simulink model "SUPERCAPACITOR_closed_loop_boost"  (R2021a)
settings: Solver=VariableStepAuto  StartTime=0.0  StopTime=10.0  RelTol=1e-3
libraries: spsSeriesRLCBranchLib x7, spsMosfetLib x4, simulink x1, spsSupercapacitorLib x1, spsVoltageMeasurementLib x1, spspowerguiLib x1
settings Model: Creator=Bhargava  LastModifiedBy=Bhargava

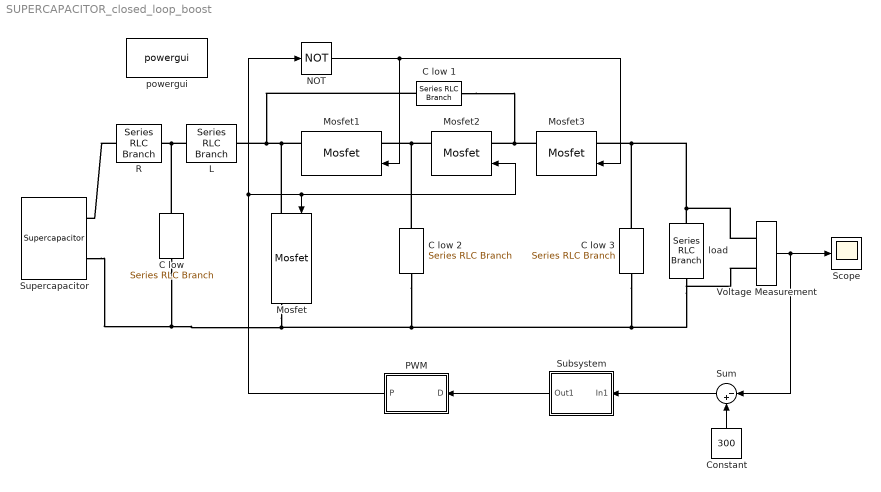
== system SUPERCAPACITOR_closed_loop_boost ==
  C low {,1..3} (4 alike) : spsSeriesRLCBranchLib/Series RLC Branch  LConnTagsString=__new0  RConnTagsString=__new0  BranchType=C  Resistance=1  Inductance=1e-3  SetiL0=off  InitialCurrent=0  Capacitance=520e-6  Setx0=off  InitialVoltage=0  Measurements=None
  Constant : Constant  Value=300
  L : spsSeriesRLCBranchLib/Series RLC Branch  LConnTagsString=__new0  RConnTagsString=__new0  BranchType=L  Resistance=1  Inductance=353e-3  SetiL0=off  InitialCurrent=0  Capacitance=1e-6  Setx0=off  InitialVoltage=0  Measurements=None
  Mosfet{,1..3} (4 alike) : spsMosfetLib/Mosfet  Ron=0.1  Lon=0  Rd=0.01  Vfd=0  IC=0  Rs=1e5  Cs=inf  Measurements=on
  NOT : Logic  Operator=NOT  IconShape=distinctive  AllPortsSameDT=off  OutDataTypeStr=boolean
  "PWM " : Subsystem
  R : spsSeriesRLCBranchLib/Series RLC Branch  LConnTagsString=__new0  RConnTagsString=__new0  BranchType=R  Resistance=0.0001  Inductance=1e-3  SetiL0=off  InitialCurrent=0  Capacitance=1e-6  Setx0=off  InitialVoltage=0  Measurements=None
  Scope : Scope
  Subsystem : Subsystem
  Sum : Sum  Inputs=|-+
  Supercapacitor : spsSupercapacitorLib/Supercapacitor  C=99.5  Rdc=8.9e-3  Voltage=200  Ns=18  Np=1  Vinit=45  Temp=25  PresetModel=off  EstParam=off  Nc=1  r=1e-9  epsilon=6.0208e-10  Ich=10  Vstern="[0.161  2.7  7.8]"  Self_dis=on  Ioc=10  Vself="[48  47.8  47.06  44.65]"  demandeplot=off  I="[10  20 100  500]"  Units=sec  Vmax=0  If=0  deltaV=0  alpha=0  sec=0
      settings: SourceProductBaseCode=PS
  Voltage Measurement : spsVoltageMeasurementLib/Voltage Measurement  PhasorSimulation=off  OutputType=Complex  PSBequivalent=0
  load : spsSeriesRLCBranchLib/Series RLC Branch  LConnTagsString=__new0  RConnTagsString=__new0  BranchType=R  Resistance=300  Inductance=1e-3  SetiL0=off  InitialCurrent=0  Capacitance=1e-6  Setx0=off  InitialVoltage=0  Measurements=None
  powergui : spspowerguiLib/powergui  Priority=1  SimulationMode=Discrete  SampleTime=2e-6  frequency=60  Iterations=50  frequencyindice=0  Pbase=100e6  ErrMax=1e-4  UnitsV=kV  UnitsW=MW  buscounter=0  FunctionMessages=off  echomessages=off  EnableUseOfTLC=off  CurrentSourceSwitches=off  DisableSnubberDevices=off  DisableRonSwitches=off  DisableVfSwitches=off  DisplayEquations=off  AutomaticDiscreteSolvers=off  SolverType=Tustin/Backward Euler (TBE)  Interpol=off  ExternalGateDelay=off  methode=off  Ts=100  x0status=blocks  SPID=on  SwTol=0  HookPort=off  NonlinearTolerance=1e-4  nMaxIteration=100  ContinueOnMaxIteration=off  RestoreLinks=warning  ResistiveCurrentMeasurement=off  Frange=[0:2:500]  Ylog=off  Xlog=on  ShowGrid=off  save=off  variable=ZData  structure=0  ZoomFFT=off  StartTime=0.0  cycles=1  DisplayStyle=1  fundamental=60  FreqAxis=off  MaxFrequency=1000  frequencyindicesteady=1  RmsSteady=1  display=off
  wires:
  Voltage Measurement/1 -> Sum/1, Scope/1
  NOT/1 -> Mosfet3/1, Mosfet1/1
  Constant/1 -> Sum/2
  "PWM "/1(P) -> NOT/1, Mosfet2/1, Mosfet/1
  Sum/1 -> Subsystem/1(In1)
  Subsystem/1(Out1) -> "PWM "/1(D)
  connections:
  load/LConn1 -- Voltage Measurement/LConn1 -- C low 3/LConn1 -- Mosfet3/LConn1
  L/LConn1 -- R/RConn1 -- "C low "/LConn1
  R/LConn1 -- Supercapacitor/LConn1
  Supercapacitor/LConn2 -- Voltage Measurement/LConn2 -- load/RConn1 -- C low 3/RConn1 -- C low 2/RConn1 -- Mosfet/RConn1 -- "C low "/RConn1
  Mosfet/LConn1 -- L/RConn1 -- C low 1/RConn1 -- Mosfet1/RConn1
  Mosfet2/RConn1 -- C low 2/LConn1 -- Mosfet1/LConn1
  Mosfet3/RConn1 -- C low 1/LConn1 -- Mosfet2/LConn1

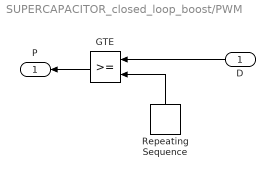
== system SUPERCAPACITOR_closed_loop_boost/PWM  ==
  D : Inport
  GTE : RelationalOperator  OutDataTypeStr=boolean  RndMeth=Simplest
  Repeating Sequence : simulink/Sources/Repeating Sequence  rep_seq_t=[0 1/20e3]  rep_seq_y=[0 1]
  P : Outport
  wires:
  GTE/1 -> P/1
  Repeating Sequence/1 -> GTE/2
  D/1 -> GTE/1

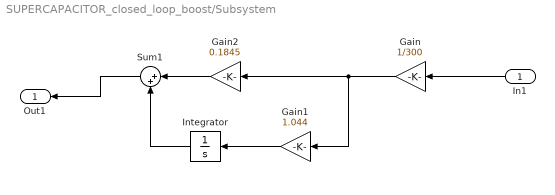
== system SUPERCAPACITOR_closed_loop_boost/Subsystem ==
  In1 : Inport
  Gain : Gain  Gain=1/300
  Gain1 : Gain  Gain=1.044
  Gain2 : Gain  Gain=0.1845
  Integrator : Integrator
  Sum1 : Sum  Inputs=|++
  Out1 : Outport
  wires:
  In1/1 -> Gain/1
  Sum1/1 -> Out1/1
  Gain1/1 -> Integrator/1
  Integrator/1 -> Sum1/2
  Gain/1 -> Gain1/1, Gain2/1
  Gain2/1 -> Sum1/1
